simulink model "bh_test_XLSREAD"  (R2016a)
settings: Solver=ode45  StartTime=0.0  StopTime=30  RelTol=1e-5
libraries: simulink x2
settings Model: Creator=bhorton  LastModifiedBy=bhorton

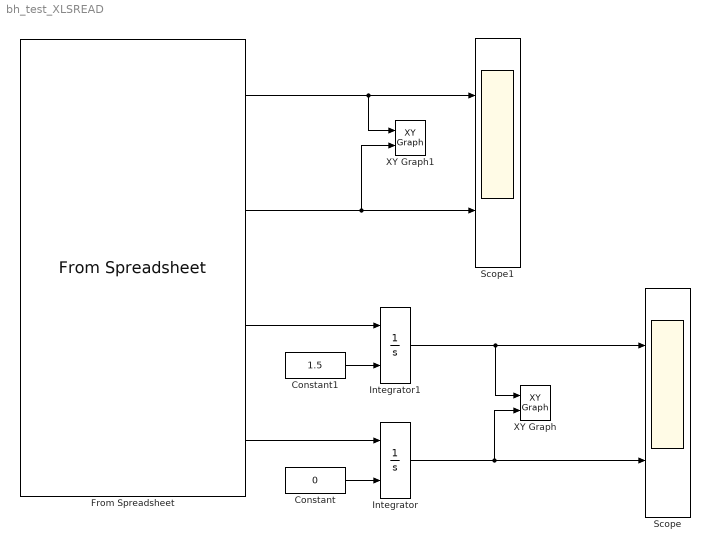
== system bh_test_XLSREAD ==
  Constant : Constant  Value=0
  Constant1 : Constant  Value=1.5
  From Spreadsheet : FromSpreadsheet  FileName=bh_hello_complete.xlsx  SheetName=COMP_SPLINE  SampleTime=0.01  ExtrapolationBeforeFirstDataPoint=Hold first value  ExtrapolationAfterLastDataPoint=Hold last value
  Integrator : Integrator  InitialConditionSource=external
  Integrator1 : Integrator  InitialConditionSource=external
  Scope : Scope  NumInputPorts=2
  Scope1 : Scope  NumInputPorts=2
  XY Graph : simulink/Sinks/XY Graph  xmin=-2  xmax=2  ymin=-2  ymax=2  st=-1
  XY Graph1 : simulink/Sinks/XY Graph  xmin=-2  xmax=2  ymin=-2  ymax=2  st=-1
  wires:
  Constant/1 -> Integrator/2
  From Spreadsheet/4 -> Integrator/1
  Constant1/1 -> Integrator1/2
  From Spreadsheet/3 -> Integrator1/1
  Integrator1/1 -> XY Graph/1, Scope/1
  Integrator/1 -> XY Graph/2, Scope/2
  From Spreadsheet/1 -> XY Graph1/1, Scope1/1
  From Spreadsheet/2 -> XY Graph1/2, Scope1/2
